simulink model "sim1"  (R2024a)
settings: Solver=FixedStepAuto  StartTime=0.0  StopTime=20.0  FixedStep=1e-3  RelTol=1e-3
settings Model: Creator=alexe  LastModifiedBy=alexe

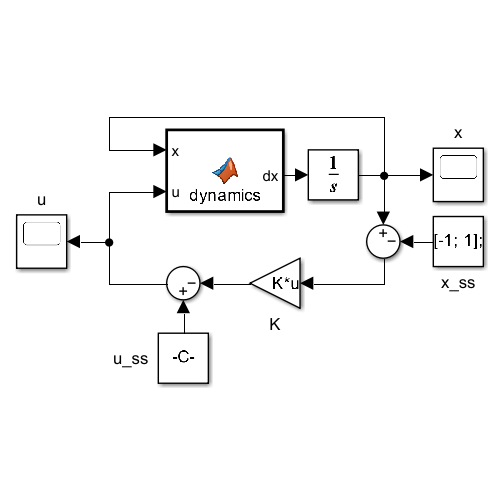
[thumbnail: Simulink's stored preview of the top-level diagram]
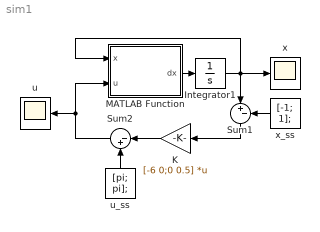
== system sim1 ==
  Integrator1 : Integrator  InitialCondition=[-0.9; 1.1];
  K : Gain  Gain=[-6 0;0 0.5]  Multiplication=Matrix(K*u)
  MATLAB Function : MATLAB Function  TreatAsAtomicUnit=on
  Sum1 : Sum  Inputs=|+-
  Sum2 : Sum  Inputs=|-+
  u : Scope
  u_ss : Constant  Value=[pi; pi];  VectorParams1D=off
  x : Scope
  x_ss : Constant  Value=[-1; 1];  VectorParams1D=off
  wires:
  K/1 -> Sum2/1
  Sum1/1 -> K/1
  x_ss/1 -> Sum1/2
  u_ss/1 -> Sum2/2
  MATLAB Function/1(dx) -> Integrator1/1
  Integrator1/1 -> Sum1/1, MATLAB Function/1(x), x/1
  Sum2/1 -> MATLAB Function/2(u), u/1

== matlab function sim1/MATLAB Function ==
  data: x input; u input; dx output
function dx = dynamics(x, u)
    x1 = x(1);
    x2 = x(2);

    u1= u(1);
    u2 = u(2);

    dx = zeros(2,1);
    dx(1) = -x1+2*x1^3+x2+sin(u1);
    dx(2) = -x1-x2+3*sin(u2);
end
